simulink model "sampleModel1825_4_sub"  (R2023a)
settings: Solver=VariableStepAuto  StartTime=0.0  StopTime=10.0  RelTol=1e-3
libraries: hdlsllib x2, simulink x1
settings Model: Creator=user1  LastModifiedBy=user1
settings OptimizationCC: BlockReduction=off  ConditionallyExecuteInputs=off

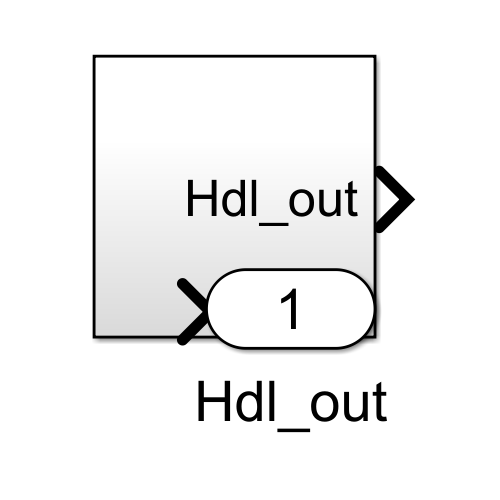
[thumbnail: Simulink's stored preview of the top-level diagram]
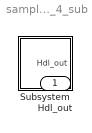
== system sampleModel1825_4_sub ==
  Subsystem : Subsystem
  Hdl_out : Outport  OutDataTypeStr=uint8

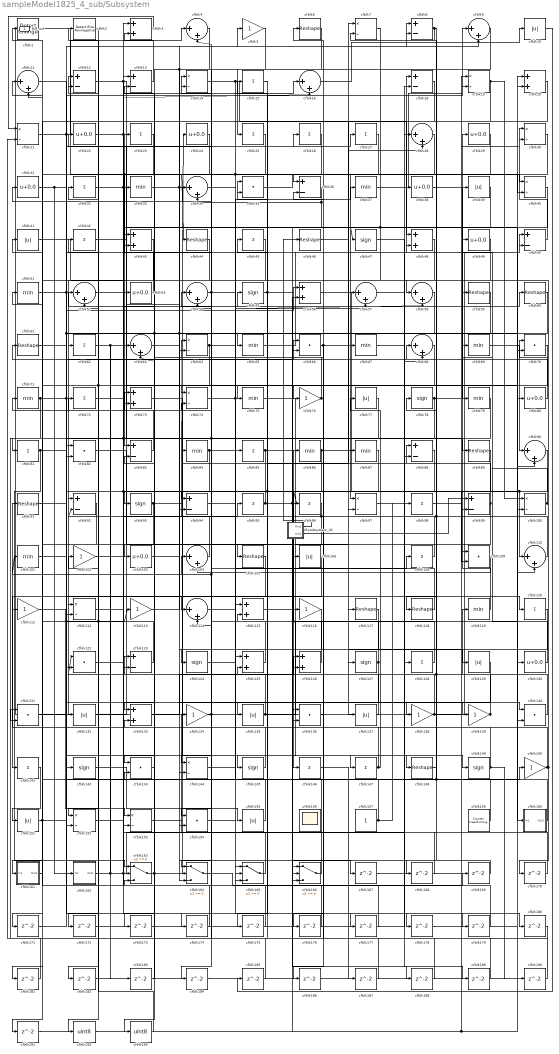
== system sampleModel1825_4_sub/Subsystem ==
  Mysubsystem_34 : Subsystem  TreatAsAtomicUnit=on  RTWFcnName=Mysubsystem_34
      settings: RTWFcnNameOpts=User specified  RTWFileNameOpts=Use function name
  cfblk1 : simulink/Logic and Bit Operations/Detect Change  vinit=0  OutDataTypeStr=uint8
      settings: LibrarySourceBlock=|
      | hdlsllib/Logic and Bit
      | Operations/Detect
      | Change
  cfblk{10,39,41,77,106,129,132,135,137,151,155} (11 alike) : Abs  OutDataTypeStr=uint8  SaturateOnIntegerOverflow=off
  cfblk{7,14,19,21,30,40,64,74,97,100,112,144,152..153} (14 alike) : Product  Inputs=*/  OutDataTypeStr=uint8  RndMeth=Zero  SaturateOnIntegerOverflow=on
  cfblk{33,37,51,65,67,69,71,75,79,84,86..87,101,119} (14 alike) : MinMax  OutDataTypeStr=uint8
  cfblk{5,76,102,111,113,116,134,138..139,150} (10 alike) : Gain  OutDataTypeStr=uint8
  cfblk{22,24,29,31,38,49,53,80,103,130} (10 alike) : Bias  Bias=0.0  SaturateOnIntegerOverflow=off
  cfblk{4,9,11,16,28,34,52,54,57..58,63,68,90,104,110,114} (16 alike) : Sum  Inputs=|++  OutDataTypeStr=uint8
  cfblk{6,44,46,59..61,89,91,105,117..118,148} (12 alike) : Reshape
  cfblk{15,23,25..27,32,42,45,62,72,81,85,95..96,98,108,120,128,141,146..147} (21 alike) : Sum  Inputs=+  OutDataTypeStr=uint8
  cfblk{35,66,70,82,109,122,131,136,140,143,154} (11 alike) : DotProduct  OutDataTypeStr=uint8
  cfblk{3,20,43,48,56,73,115,125..126,133} (10 alike) : Sum  OutDataTypeStr=uint8
  cfblk{8,12..13,18,36,50,83,88,92,94,99,123} (12 alike) : Sum  Inputs=+-  OutDataTypeStr=uint8
  cfblk{47,55,78,93,124,127,142,145,149} (9 alike) : Signum
  cfblk156 : Scope
      settings: Floating=on
  cfblk157 : Constant  OutDataTypeStr=uint8  SampleTime=-1
  cfblk159 : hdlsllib/Sources/Counter Free-Running  NumBits=16  tsamp=-1
  cfblk160 : Subsystem
      settings: LibrarySourceBlock=|
      | hdlsllib/Ports &
      | Subsystems/Subsystem
  cfblk161 : Subsystem
      settings: LibrarySourceBlock=|
      | hdlsllib/Ports &
      | Subsystems/Subsystem
  cfblk162 : Subsystem
      settings: LibrarySourceBlock=|
      | hdlsllib/Ports &
      | Subsystems/Subsystem
  cfblk{163..166} (4 alike) : Switch  OutDataTypeStr=uint8  SaturateOnIntegerOverflow=off  InputSameDT=off
  cfblk{167..191} (25 alike) : Delay  SampleTime=1
  cfblk192 : DataTypeConversion  OutDataTypeStr=uint8  SaturateOnIntegerOverflow=off  RndMeth=Floor
  cfblk193 : DataTypeConversion  OutDataTypeStr=uint8  SaturateOnIntegerOverflow=off  RndMeth=Floor
  cfblk2 : hdlsllib/Logic and Bit Operations/Detect Rise Nonnegative  vinit=0  OutDataTypeStr=uint8
  Hdl_out : Outport  OutDataTypeStr=uint8
  wires:
  cfblk50/1 -> cfblk30/1
  cfblk157/1 -> cfblk51/1, cfblk98/1
  cfblk148/1 -> cfblk78/1
  cfblk60/1 -> cfblk132/1
  cfblk16/1 -> cfblk10/1
  cfblk70/1 -> cfblk172/1, cfblk171/1
  cfblk59/1 -> cfblk94/2, cfblk63/2, cfblk112/1
  cfblk100/1 -> cfblk49/1, cfblk58/1
  cfblk111/1 -> cfblk153/1
  cfblk1/1 -> cfblk36/1
  cfblk163/1 -> cfblk143/2, cfblk55/1
  cfblk132/1 -> cfblk27/1
  cfblk73/1 -> cfblk145/1
  cfblk165/1 -> cfblk134/1
  cfblk92/1 -> cfblk112/2
  cfblk2/1 -> cfblk192/1
  cfblk79/1 -> cfblk173/1, cfblk144/1
  cfblk138/1 -> cfblk35/1, cfblk50/1
  cfblk24/1 -> cfblk191/1, cfblk83/1
  cfblk150/1 -> cfblk35/2, cfblk170/1, cfblk70/1
  cfblk27/1 -> cfblk97/1
  cfblk54/1 -> cfblk14/1, cfblk125/1
  cfblk131/1 -> cfblk50/2, cfblk113/1
  cfblk119/1 -> cfblk29/1
  cfblk99/1 -> cfblk126/2, cfblk45/1
  cfblk110/1 -> cfblk8/2, cfblk24/1
  cfblk65/1 -> cfblk18/1
  cfblk75/1 -> cfblk148/1
  cfblk80/1 -> cfblk61/1
  cfblk89/1 -> cfblk146/1
  cfblk160/1(Out1) -> cfblk64/1
  cfblk87/1 -> cfblk133/1
  cfblk22/1 -> cfblk16/2, cfblk127/1, cfblk88/2, cfblk136/2, cfblk96/1
  cfblk12/1 -> cfblk40/2, cfblk76/1
  cfblk57/1 -> cfblk149/1
  cfblk128/1 -> cfblk86/1, cfblk43/2, cfblk101/1
  cfblk64/1 -> cfblk59/1, cfblk82/2
  cfblk127/1 -> cfblk154/2, cfblk73/1
  cfblk44/1 -> cfblk62/1
  cfblk142/1 -> cfblk155/1
  cfblk5/1 -> cfblk25/1
  cfblk42/1 -> cfblk160/1(In1)
  cfblk38/1 -> cfblk79/1
  cfblk162/1(Out1) -> cfblk63/1, cfblk16/1, cfblk18/2
  cfblk20/1 -> cfblk84/1
  cfblk9/1 -> cfblk103/1
  cfblk56/1 -> cfblk128/1
  cfblk81/1 -> cfblk120/1, cfblk163/1
  cfblk152/1 -> cfblk95/1
  cfblk21/1 -> cfblk87/1, cfblk4/1
  cfblk28/1 -> cfblk64/2
  cfblk159/1 -> cfblk115/2, cfblk88/1
  cfblk69/1 -> cfblk90/1
  cfblk26/1 -> cfblk165/3, cfblk44/1
  cfblk86/1 -> cfblk109/2, cfblk165/2, cfblk105/1
  cfblk82/1 -> cfblk116/1
  cfblk153/1 -> cfblk115/1
  cfblk106/1 -> cfblk141/1
  cfblk139/1 -> Hdl_out/1, cfblk68/1, cfblk122/1
  cfblk85/1 -> cfblk93/1, cfblk89/1
  cfblk49/1 -> cfblk92/1
  cfblk134/1 -> cfblk184/1, cfblk4/2
  cfblk130/1 -> cfblk69/1
  cfblk115/1 -> cfblk108/1
  cfblk93/1 -> cfblk7/1, cfblk152/1
  cfblk76/1 -> cfblk6/1, cfblk52/1
  cfblk90/1 -> cfblk168/1, cfblk110/1
  cfblk145/1 -> cfblk91/1
  cfblk23/1 -> cfblk122/2
  cfblk155/1 -> cfblk32/1
  cfblk52/1 -> cfblk137/1
  cfblk19/1 -> cfblk100/1, cfblk97/2
  cfblk135/1 -> cfblk114/2, cfblk20/1
  cfblk166/1 -> cfblk54/1
  cfblk126/1 -> cfblk71/1
  cfblk141/1 -> cfblk151/1
  cfblk37/1 -> cfblk9/1
  cfblk140/1 -> cfblk119/1
  cfblk68/1 -> cfblk163/2
  cfblk94/1 -> cfblk140/1
  cfblk41/1 -> cfblk53/1
  cfblk14/1 -> cfblk180/1, cfblk48/1
  cfblk104/1 -> cfblk72/1
  cfblk31/1 -> cfblk162/1(In1), cfblk26/1
  cfblk123/1 -> cfblk11/2, cfblk102/1
  cfblk84/1 -> cfblk193/1, cfblk57/2
  cfblk8/1 -> cfblk7/2, cfblk138/1
  cfblk149/1 -> cfblk190/1, cfblk42/1
  cfblk125/1 -> cfblk22/1
  cfblk151/1 -> cfblk41/1, cfblk150/1
  cfblk11/1 -> cfblk177/1, cfblk70/2
  cfblk108/1 -> cfblk66/1
  cfblk3/1 -> cfblk21/1
  cfblk78/1 -> cfblk153/2, cfblk30/2
  cfblk40/1 -> cfblk65/1
  cfblk117/1 -> cfblk144/2
  cfblk35/1 -> cfblk38/1
  cfblk137/1 -> cfblk13/2
  cfblk36/1 -> cfblk34/2, cfblk166/3
  cfblk114/1 -> cfblk37/1
  cfblk102/1 -> cfblk60/1
  cfblk15/1 -> cfblk135/1
  cfblk116/1 -> cfblk124/1
  cfblk143/1 -> cfblk123/1
  cfblk51/1 -> cfblk8/1, cfblk147/1
  cfblk129/1 -> cfblk164/1
  cfblk61/1 -> cfblk142/1
  cfblk13/1 -> cfblk3/2
  cfblk83/1 -> cfblk12/1
  cfblk45/1 -> cfblk111/1
  cfblk58/1 -> cfblk75/1
  cfblk63/1 -> cfblk136/1
  cfblk109/1 -> cfblk104/2
  cfblk30/1 -> cfblk118/1
  cfblk122/1 -> cfblk9/2
  cfblk124/1 -> cfblk106/1
  cfblk43/1 -> cfblk52/2
  cfblk77/1 -> cfblk81/1
  cfblk66/1 -> cfblk186/1, cfblk129/1
  cfblk98/1 -> cfblk39/1
  cfblk101/1 -> cfblk66/2
  cfblk105/1 -> cfblk154/1
  cfblk147/1 -> cfblk133/2, cfblk77/1
  cfblk33/1 -> cfblk40/1, cfblk80/1
  cfblk53/1 -> cfblk23/1
  cfblk97/1 -> cfblk28/1
  cfblk48/1 -> cfblk114/1
  cfblk120/1 -> cfblk164/2
  cfblk74/1 -> cfblk58/2, cfblk85/1
  cfblk118/1 -> cfblk31/1
  cfblk7/1 -> cfblk57/1, cfblk47/1
  cfblk113/1 -> cfblk34/1
  cfblk88/1 -> cfblk152/2
  cfblk95/1 -> cfblk94/1, cfblk188/1, cfblk117/1
  cfblk6/1 -> cfblk74/1
  cfblk144/1 -> cfblk48/2
  cfblk46/1 -> cfblk28/2
  cfblk72/1 -> cfblk139/1
  cfblk91/1 -> cfblk56/1
  cfblk39/1 -> cfblk43/1
  cfblk32/1 -> cfblk14/2, cfblk67/1
  cfblk55/1 -> cfblk100/2, cfblk15/1
  cfblk25/1 -> cfblk182/1, cfblk33/1
  cfblk4/1 -> cfblk143/1, cfblk164/3
  cfblk154/1 -> cfblk165/1
  cfblk161/1(Out1) -> cfblk11/1
  cfblk62/1 -> cfblk183/1, cfblk5/1
  cfblk71/1 -> cfblk131/2, cfblk140/2, cfblk19/2
  cfblk133/1 -> cfblk126/1
  cfblk96/1 -> cfblk161/1(In1), cfblk92/2
  cfblk103/1 -> cfblk167/1
  cfblk167/1 -> cfblk109/1
  cfblk168/1 -> cfblk104/1
  cfblk164/1 -> cfblk169/1
  cfblk169/1 -> cfblk166/2
  cfblk170/1 -> cfblk13/1
  cfblk171/1 -> cfblk82/1
  cfblk172/1 -> cfblk68/2
  cfblk173/1 -> cfblk123/2
  cfblk112/1 -> cfblk174/1
  cfblk174/1 -> cfblk1/1
  cfblk29/1 -> cfblk175/1
  cfblk175/1 -> cfblk54/2
  cfblk136/1 -> cfblk176/1
  cfblk176/1 -> cfblk73/2
  cfblk177/1 -> cfblk3/1
  cfblk34/1 -> cfblk178/1
  cfblk178/1 -> cfblk90/2
  cfblk67/1 -> cfblk179/1
  cfblk179/1 -> cfblk83/2
  cfblk180/1 -> cfblk21/2
  cfblk18/1 -> cfblk181/1
  cfblk181/1 -> cfblk131/1
  cfblk182/1 -> cfblk110/2
  cfblk183/1 -> cfblk163/3
  cfblk184/1 -> cfblk20/2
  cfblk10/1 -> cfblk185/1
  cfblk185/1 -> cfblk12/2
  cfblk186/1 -> cfblk19/1
  cfblk146/1 -> cfblk187/1
  cfblk187/1 -> cfblk166/1
  cfblk188/1 -> cfblk74/2
  cfblk47/1 -> cfblk189/1
  cfblk189/1 -> cfblk36/2
  cfblk190/1 -> cfblk125/2
  cfblk191/1 -> cfblk56/2
  cfblk192/1 -> cfblk130/1, cfblk99/2
  cfblk193/1 -> cfblk2/1
  Mysubsystem_34/1(Out1) -> cfblk46/1
  Mysubsystem_34/2(Out2) -> cfblk99/1

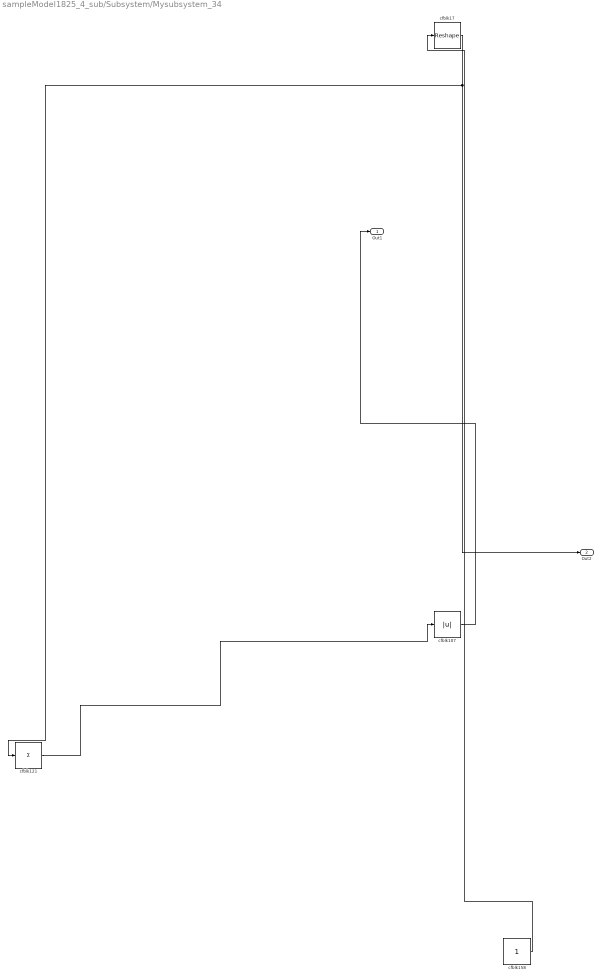
== system sampleModel1825_4_sub/Subsystem/Mysubsystem_34 ==
  cfblk107 : Abs  SaturateOnIntegerOverflow=off
  cfblk121 : Sum  Inputs=+
  cfblk158 : Constant  SampleTime=-1
  cfblk17 : Reshape
  Out1 : Outport
  Out2 : Outport  Port=2
  wires:
  cfblk107/1 -> Out1/1
  cfblk158/1 -> cfblk17/1
  cfblk121/1 -> cfblk107/1
  cfblk17/1 -> cfblk121/1, Out2/1

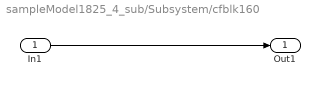
== system sampleModel1825_4_sub/Subsystem/cfblk160 ==
  In1 : Inport
  Out1 : Outport
  wires:
  In1/1 -> Out1/1

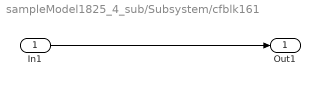
== system sampleModel1825_4_sub/Subsystem/cfblk161 ==
  In1 : Inport
  Out1 : Outport
  wires:
  In1/1 -> Out1/1

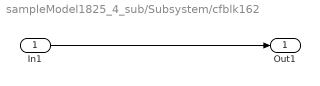
== system sampleModel1825_4_sub/Subsystem/cfblk162 ==
  In1 : Inport
  Out1 : Outport
  wires:
  In1/1 -> Out1/1
